simulink model "StPassCmprtMdCrtMdStat"  (R2018b)
settings: Solver=FixedStepDiscrete  StartTime=0.0  StopTime=10.0  FixedStep=0.01  RelTol=1e-3
settings Model: Creator=sn2xws  LastModifiedBy=sn2xws
settings DataIOCC: SaveFormat=StructureWithTime
settings OptimizationCC: DefaultParameterBehavior=Inlined  EnhancedBackFolding=on  PassReuseOutputArgsAs=Individual arguments  ZeroExternalMemoryAtStartup=off  ZeroInternalMemoryAtStartup=off  OptimizeBlockOrder=speed  DifferentSizesBufferReuse=on  OptimizationCustomize=off
settings DebuggingCC: ParameterTunabilityLossMsg=error
settings ModelReferenceCC: ModelReferenceNumInstancesAllowed=Single
settings SFSimCC: MATLABDynamicMemAlloc=off
settings RTWCC: SystemTargetFile=autosar.tlc  GenCodeOnly=on  TemplateMakefile=ert_default_tmf  Description=AUTOSAR  GenerateReport=on  IncludeHyperlinkInReport=on  LaunchReport=on  GenerateTraceInfo=on  GenerateTraceReport=on  GenerateTraceReportSl=on  GenerateTraceReportSf=on  GenerateTraceReportEml=on
settings CodeAppCC: ForceParamTrailComments=on  IgnoreCustomStorageClasses=off  OperatorAnnotations=on  SimulinkDataObjDesc=on  SFDataObjDesc=on  InsertBlockDesc=on
settings STFCustomTargetCC: TargetLangStandard=C99 (ISO)  MultiwordLength=256  ParMdlRefBuildCompliant=on  CompOptLevelCompliant=on  IncludeMdlTerminateFcn=off  CombineOutputUpdateFcns=on  SuppressErrorStatus=on  ERTCustomFileBanners=on  SupportNonFinite=off  SupportComplex=off  SupportContinuousTime=off  SupportNonInlinedSFcns=off  RemoveResetFunc=on  MATLABClassNameForMDSCustomization=Simulink.SoftwareTarget.ERTCustomization  AutosarCompliant=on  UseToolchainInfoCompliant=on  LookupTableObjectStructAxisOrder=2,1,3,4,...  LUTObjectStructOrderEvenSpacing=Size,Table,Breakpoints  SystemTargetFile=autosar.tlc
settings ERTTargetCC: TargetLangStandard=C99 (ISO)  ConcurrentExecutionCompliant=off  IncludeMdlTerminateFcn=off  SuppressErrorStatus=on  SupportNonFinite=off  SupportComplex=off  ModelStepFunctionPrototypeControlCompliant=off  CPPClassGenCompliant=off  AutosarCompliant=on  LookupTableObjectStructAxisOrder=2,1,3,4,...  LUTObjectStructOrderEvenSpacing=Size,Table,Breakpoints  InlinedParameterPlacement=NonHierarchical  ERTCustomFileTemplate=example_file_process.tlc

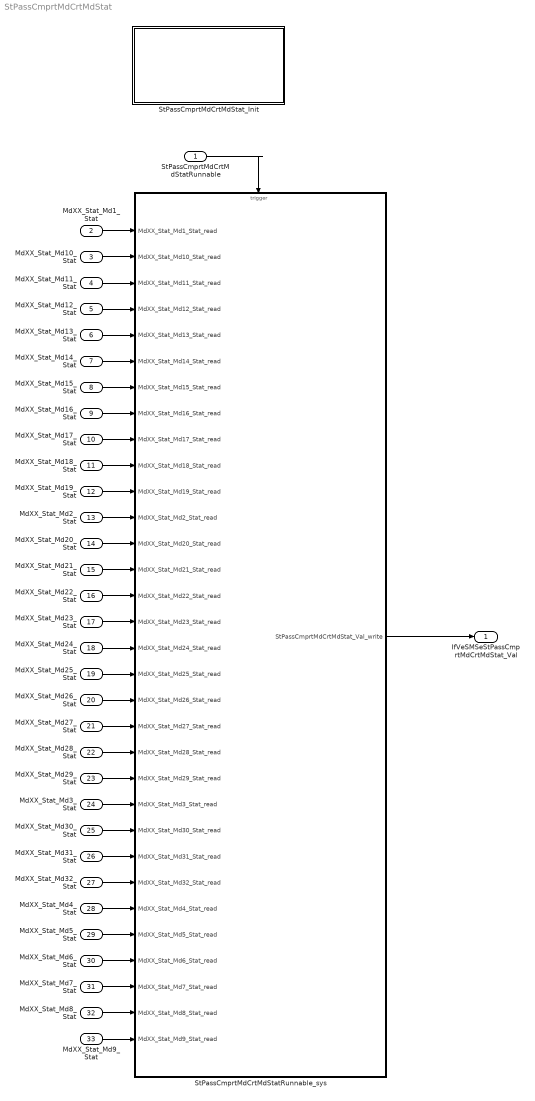
== system StPassCmprtMdCrtMdStat ==
  StPassCmprtMdCrtMdStatRunnable : Inport  SampleTime=0.01  OutputFunctionCall=on
  MdXX_Stat_Md1_Stat : Inport  Port=2  OutDataTypeStr=uint8  PortDimensions=1
  MdXX_Stat_Md10_Stat : Inport  Port=3  OutDataTypeStr=uint8  PortDimensions=1
  MdXX_Stat_Md11_Stat : Inport  Port=4  OutDataTypeStr=uint8  PortDimensions=1
  MdXX_Stat_Md12_Stat : Inport  Port=5  OutDataTypeStr=uint8  PortDimensions=1
  MdXX_Stat_Md13_Stat : Inport  Port=6  OutDataTypeStr=uint8  PortDimensions=1
  MdXX_Stat_Md14_Stat : Inport  Port=7  OutDataTypeStr=uint8  PortDimensions=1
  MdXX_Stat_Md15_Stat : Inport  Port=8  OutDataTypeStr=uint8  PortDimensions=1
  MdXX_Stat_Md16_Stat : Inport  Port=9  OutDataTypeStr=uint8  PortDimensions=1
  MdXX_Stat_Md17_Stat : Inport  Port=10  OutDataTypeStr=uint8  PortDimensions=1
  MdXX_Stat_Md18_Stat : Inport  Port=11  OutDataTypeStr=uint8  PortDimensions=1
  MdXX_Stat_Md19_Stat : Inport  Port=12  OutDataTypeStr=uint8  PortDimensions=1
  MdXX_Stat_Md2_Stat : Inport  Port=13  OutDataTypeStr=uint8  PortDimensions=1
  MdXX_Stat_Md20_Stat : Inport  Port=14  OutDataTypeStr=uint8  PortDimensions=1
  MdXX_Stat_Md21_Stat : Inport  Port=15  OutDataTypeStr=uint8  PortDimensions=1
  MdXX_Stat_Md22_Stat : Inport  Port=16  OutDataTypeStr=uint8  PortDimensions=1
  MdXX_Stat_Md23_Stat : Inport  Port=17  OutDataTypeStr=uint8  PortDimensions=1
  MdXX_Stat_Md24_Stat : Inport  Port=18  OutDataTypeStr=uint8  PortDimensions=1
  MdXX_Stat_Md25_Stat : Inport  Port=19  OutDataTypeStr=uint8  PortDimensions=1
  MdXX_Stat_Md26_Stat : Inport  Port=20  OutDataTypeStr=uint8  PortDimensions=1
  MdXX_Stat_Md27_Stat : Inport  Port=21  OutDataTypeStr=uint8  PortDimensions=1
  MdXX_Stat_Md28_Stat : Inport  Port=22  OutDataTypeStr=uint8  PortDimensions=1
  MdXX_Stat_Md29_Stat : Inport  Port=23  OutDataTypeStr=uint8  PortDimensions=1
  MdXX_Stat_Md3_Stat : Inport  Port=24  OutDataTypeStr=uint8  PortDimensions=1
  MdXX_Stat_Md30_Stat : Inport  Port=25  OutDataTypeStr=uint8  PortDimensions=1
  MdXX_Stat_Md31_Stat : Inport  Port=26  OutDataTypeStr=uint8  PortDimensions=1
  MdXX_Stat_Md32_Stat : Inport  Port=27  OutDataTypeStr=uint8  PortDimensions=1
  MdXX_Stat_Md4_Stat : Inport  Port=28  OutDataTypeStr=uint8  PortDimensions=1
  MdXX_Stat_Md5_Stat : Inport  Port=29  OutDataTypeStr=uint8  PortDimensions=1
  MdXX_Stat_Md6_Stat : Inport  Port=30  OutDataTypeStr=uint8  PortDimensions=1
  MdXX_Stat_Md7_Stat : Inport  Port=31  OutDataTypeStr=uint8  PortDimensions=1
  MdXX_Stat_Md8_Stat : Inport  Port=32  OutDataTypeStr=uint8  PortDimensions=1
  MdXX_Stat_Md9_Stat : Inport  Port=33  OutDataTypeStr=uint8  PortDimensions=1
  StPassCmprtMdCrtMdStatRunnable_sys : Subsystem
  StPassCmprtMdCrtMdStat_Init : Subsystem
  IfVeSMSeStPassCmprtMdCrtMdStat_Val : Outport  OutDataTypeStr=uint8  PortDimensions=1
  wires:
  MdXX_Stat_Md1_Stat/1 -> StPassCmprtMdCrtMdStatRunnable_sys/1(MdXX_Stat_Md1_Stat_read)
  MdXX_Stat_Md10_Stat/1 -> StPassCmprtMdCrtMdStatRunnable_sys/2(MdXX_Stat_Md10_Stat_read)
  MdXX_Stat_Md11_Stat/1 -> StPassCmprtMdCrtMdStatRunnable_sys/3(MdXX_Stat_Md11_Stat_read)
  MdXX_Stat_Md12_Stat/1 -> StPassCmprtMdCrtMdStatRunnable_sys/4(MdXX_Stat_Md12_Stat_read)
  MdXX_Stat_Md13_Stat/1 -> StPassCmprtMdCrtMdStatRunnable_sys/5(MdXX_Stat_Md13_Stat_read)
  MdXX_Stat_Md14_Stat/1 -> StPassCmprtMdCrtMdStatRunnable_sys/6(MdXX_Stat_Md14_Stat_read)
  MdXX_Stat_Md15_Stat/1 -> StPassCmprtMdCrtMdStatRunnable_sys/7(MdXX_Stat_Md15_Stat_read)
  MdXX_Stat_Md16_Stat/1 -> StPassCmprtMdCrtMdStatRunnable_sys/8(MdXX_Stat_Md16_Stat_read)
  MdXX_Stat_Md17_Stat/1 -> StPassCmprtMdCrtMdStatRunnable_sys/9(MdXX_Stat_Md17_Stat_read)
  MdXX_Stat_Md18_Stat/1 -> StPassCmprtMdCrtMdStatRunnable_sys/10(MdXX_Stat_Md18_Stat_read)
  MdXX_Stat_Md19_Stat/1 -> StPassCmprtMdCrtMdStatRunnable_sys/11(MdXX_Stat_Md19_Stat_read)
  MdXX_Stat_Md2_Stat/1 -> StPassCmprtMdCrtMdStatRunnable_sys/12(MdXX_Stat_Md2_Stat_read)
  MdXX_Stat_Md20_Stat/1 -> StPassCmprtMdCrtMdStatRunnable_sys/13(MdXX_Stat_Md20_Stat_read)
  MdXX_Stat_Md21_Stat/1 -> StPassCmprtMdCrtMdStatRunnable_sys/14(MdXX_Stat_Md21_Stat_read)
  MdXX_Stat_Md22_Stat/1 -> StPassCmprtMdCrtMdStatRunnable_sys/15(MdXX_Stat_Md22_Stat_read)
  MdXX_Stat_Md23_Stat/1 -> StPassCmprtMdCrtMdStatRunnable_sys/16(MdXX_Stat_Md23_Stat_read)
  MdXX_Stat_Md24_Stat/1 -> StPassCmprtMdCrtMdStatRunnable_sys/17(MdXX_Stat_Md24_Stat_read)
  MdXX_Stat_Md25_Stat/1 -> StPassCmprtMdCrtMdStatRunnable_sys/18(MdXX_Stat_Md25_Stat_read)
  MdXX_Stat_Md26_Stat/1 -> StPassCmprtMdCrtMdStatRunnable_sys/19(MdXX_Stat_Md26_Stat_read)
  MdXX_Stat_Md27_Stat/1 -> StPassCmprtMdCrtMdStatRunnable_sys/20(MdXX_Stat_Md27_Stat_read)
  MdXX_Stat_Md28_Stat/1 -> StPassCmprtMdCrtMdStatRunnable_sys/21(MdXX_Stat_Md28_Stat_read)
  MdXX_Stat_Md29_Stat/1 -> StPassCmprtMdCrtMdStatRunnable_sys/22(MdXX_Stat_Md29_Stat_read)
  MdXX_Stat_Md3_Stat/1 -> StPassCmprtMdCrtMdStatRunnable_sys/23(MdXX_Stat_Md3_Stat_read)
  MdXX_Stat_Md30_Stat/1 -> StPassCmprtMdCrtMdStatRunnable_sys/24(MdXX_Stat_Md30_Stat_read)
  MdXX_Stat_Md31_Stat/1 -> StPassCmprtMdCrtMdStatRunnable_sys/25(MdXX_Stat_Md31_Stat_read)
  MdXX_Stat_Md32_Stat/1 -> StPassCmprtMdCrtMdStatRunnable_sys/26(MdXX_Stat_Md32_Stat_read)
  MdXX_Stat_Md4_Stat/1 -> StPassCmprtMdCrtMdStatRunnable_sys/27(MdXX_Stat_Md4_Stat_read)
  MdXX_Stat_Md5_Stat/1 -> StPassCmprtMdCrtMdStatRunnable_sys/28(MdXX_Stat_Md5_Stat_read)
  MdXX_Stat_Md6_Stat/1 -> StPassCmprtMdCrtMdStatRunnable_sys/29(MdXX_Stat_Md6_Stat_read)
  MdXX_Stat_Md7_Stat/1 -> StPassCmprtMdCrtMdStatRunnable_sys/30(MdXX_Stat_Md7_Stat_read)
  MdXX_Stat_Md8_Stat/1 -> StPassCmprtMdCrtMdStatRunnable_sys/31(MdXX_Stat_Md8_Stat_read)
  MdXX_Stat_Md9_Stat/1 -> StPassCmprtMdCrtMdStatRunnable_sys/32(MdXX_Stat_Md9_Stat_read)
  StPassCmprtMdCrtMdStatRunnable_sys/1(StPassCmprtMdCrtMdStat_Val_write) -> IfVeSMSeStPassCmprtMdCrtMdStat_Val/1
  StPassCmprtMdCrtMdStatRunnable/1 -> StPassCmprtMdCrtMdStatRunnable_sys/Trigger

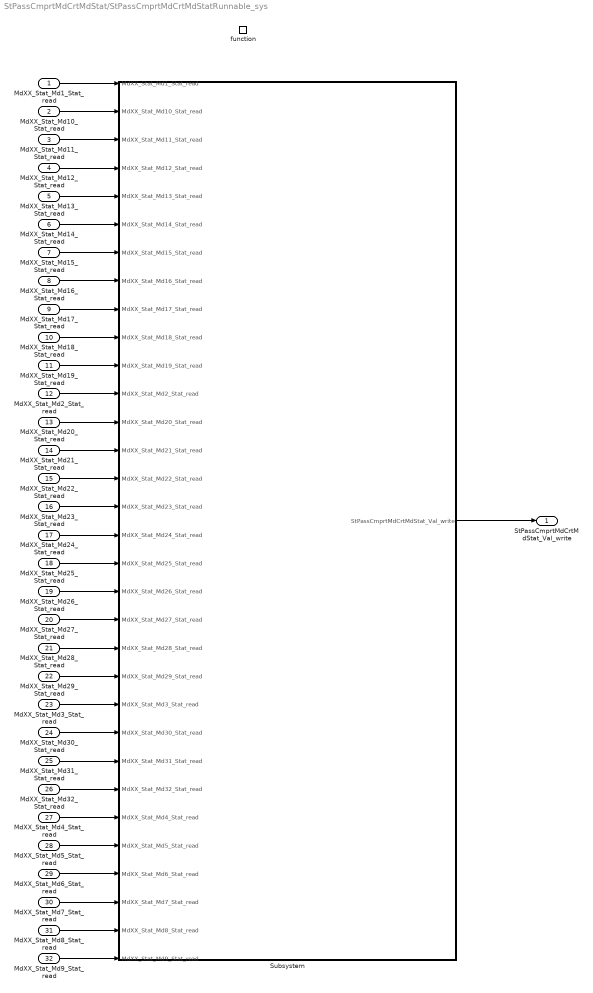
== system StPassCmprtMdCrtMdStat/StPassCmprtMdCrtMdStatRunnable_sys ==
  MdXX_Stat_Md1_Stat_read : Inport
  MdXX_Stat_Md10_Stat_read : Inport  Port=2
  MdXX_Stat_Md11_Stat_read : Inport  Port=3
  MdXX_Stat_Md12_Stat_read : Inport  Port=4
  MdXX_Stat_Md13_Stat_read : Inport  Port=5
  MdXX_Stat_Md14_Stat_read : Inport  Port=6
  MdXX_Stat_Md15_Stat_read : Inport  Port=7
  MdXX_Stat_Md16_Stat_read : Inport  Port=8
  MdXX_Stat_Md17_Stat_read : Inport  Port=9
  MdXX_Stat_Md18_Stat_read : Inport  Port=10
  MdXX_Stat_Md19_Stat_read : Inport  Port=11
  MdXX_Stat_Md2_Stat_read : Inport  Port=12
  MdXX_Stat_Md20_Stat_read : Inport  Port=13
  MdXX_Stat_Md21_Stat_read : Inport  Port=14
  MdXX_Stat_Md22_Stat_read : Inport  Port=15
  MdXX_Stat_Md23_Stat_read : Inport  Port=16
  MdXX_Stat_Md24_Stat_read : Inport  Port=17
  MdXX_Stat_Md25_Stat_read : Inport  Port=18
  MdXX_Stat_Md26_Stat_read : Inport  Port=19
  MdXX_Stat_Md27_Stat_read : Inport  Port=20
  MdXX_Stat_Md28_Stat_read : Inport  Port=21
  MdXX_Stat_Md29_Stat_read : Inport  Port=22
  MdXX_Stat_Md3_Stat_read : Inport  Port=23
  MdXX_Stat_Md30_Stat_read : Inport  Port=24
  MdXX_Stat_Md31_Stat_read : Inport  Port=25
  MdXX_Stat_Md32_Stat_read : Inport  Port=26
  MdXX_Stat_Md4_Stat_read : Inport  Port=27
  MdXX_Stat_Md5_Stat_read : Inport  Port=28
  MdXX_Stat_Md6_Stat_read : Inport  Port=29
  MdXX_Stat_Md7_Stat_read : Inport  Port=30
  MdXX_Stat_Md8_Stat_read : Inport  Port=31
  MdXX_Stat_Md9_Stat_read : Inport  Port=32
  function : TriggerPort  TriggerType=function-call  VariantControl=(inherit)  SampleTimeType=periodic  SampleTime=-1
  Subsystem : Subsystem
  StPassCmprtMdCrtMdStat_Val_write : Outport
      settings: EnsureOutportIsVirtual=on
  wires:
  MdXX_Stat_Md1_Stat_read/1 -> Subsystem/1(MdXX_Stat_Md1_Stat_read)
  MdXX_Stat_Md10_Stat_read/1 -> Subsystem/2(MdXX_Stat_Md10_Stat_read)
  MdXX_Stat_Md11_Stat_read/1 -> Subsystem/3(MdXX_Stat_Md11_Stat_read)
  MdXX_Stat_Md12_Stat_read/1 -> Subsystem/4(MdXX_Stat_Md12_Stat_read)
  MdXX_Stat_Md13_Stat_read/1 -> Subsystem/5(MdXX_Stat_Md13_Stat_read)
  MdXX_Stat_Md14_Stat_read/1 -> Subsystem/6(MdXX_Stat_Md14_Stat_read)
  MdXX_Stat_Md15_Stat_read/1 -> Subsystem/7(MdXX_Stat_Md15_Stat_read)
  MdXX_Stat_Md16_Stat_read/1 -> Subsystem/8(MdXX_Stat_Md16_Stat_read)
  MdXX_Stat_Md17_Stat_read/1 -> Subsystem/9(MdXX_Stat_Md17_Stat_read)
  MdXX_Stat_Md18_Stat_read/1 -> Subsystem/10(MdXX_Stat_Md18_Stat_read)
  MdXX_Stat_Md19_Stat_read/1 -> Subsystem/11(MdXX_Stat_Md19_Stat_read)
  MdXX_Stat_Md2_Stat_read/1 -> Subsystem/12(MdXX_Stat_Md2_Stat_read)
  MdXX_Stat_Md20_Stat_read/1 -> Subsystem/13(MdXX_Stat_Md20_Stat_read)
  MdXX_Stat_Md21_Stat_read/1 -> Subsystem/14(MdXX_Stat_Md21_Stat_read)
  MdXX_Stat_Md22_Stat_read/1 -> Subsystem/15(MdXX_Stat_Md22_Stat_read)
  MdXX_Stat_Md23_Stat_read/1 -> Subsystem/16(MdXX_Stat_Md23_Stat_read)
  MdXX_Stat_Md24_Stat_read/1 -> Subsystem/17(MdXX_Stat_Md24_Stat_read)
  MdXX_Stat_Md25_Stat_read/1 -> Subsystem/18(MdXX_Stat_Md25_Stat_read)
  MdXX_Stat_Md26_Stat_read/1 -> Subsystem/19(MdXX_Stat_Md26_Stat_read)
  MdXX_Stat_Md27_Stat_read/1 -> Subsystem/20(MdXX_Stat_Md27_Stat_read)
  MdXX_Stat_Md28_Stat_read/1 -> Subsystem/21(MdXX_Stat_Md28_Stat_read)
  MdXX_Stat_Md29_Stat_read/1 -> Subsystem/22(MdXX_Stat_Md29_Stat_read)
  MdXX_Stat_Md3_Stat_read/1 -> Subsystem/23(MdXX_Stat_Md3_Stat_read)
  MdXX_Stat_Md30_Stat_read/1 -> Subsystem/24(MdXX_Stat_Md30_Stat_read)
  MdXX_Stat_Md31_Stat_read/1 -> Subsystem/25(MdXX_Stat_Md31_Stat_read)
  MdXX_Stat_Md32_Stat_read/1 -> Subsystem/26(MdXX_Stat_Md32_Stat_read)
  MdXX_Stat_Md4_Stat_read/1 -> Subsystem/27(MdXX_Stat_Md4_Stat_read)
  MdXX_Stat_Md5_Stat_read/1 -> Subsystem/28(MdXX_Stat_Md5_Stat_read)
  MdXX_Stat_Md6_Stat_read/1 -> Subsystem/29(MdXX_Stat_Md6_Stat_read)
  MdXX_Stat_Md7_Stat_read/1 -> Subsystem/30(MdXX_Stat_Md7_Stat_read)
  MdXX_Stat_Md8_Stat_read/1 -> Subsystem/31(MdXX_Stat_Md8_Stat_read)
  MdXX_Stat_Md9_Stat_read/1 -> Subsystem/32(MdXX_Stat_Md9_Stat_read)
  Subsystem/1(StPassCmprtMdCrtMdStat_Val_write) -> StPassCmprtMdCrtMdStat_Val_write/1

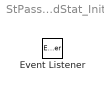
== system StPassCmprtMdCrtMdStat/StPassCmprtMdCrtMdStat_Init ==
  Event Listener : EventListener  EventName=reset

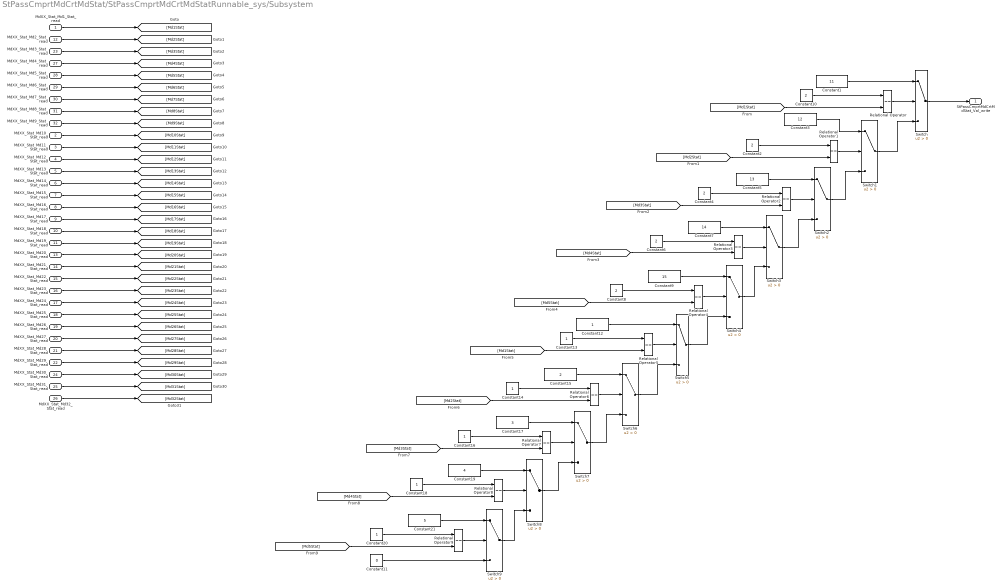
== system StPassCmprtMdCrtMdStat/StPassCmprtMdCrtMdStatRunnable_sys/Subsystem ==
  MdXX_Stat_Md1_Stat_read : Inport
  MdXX_Stat_Md10_Stat_read : Inport  Port=2
  MdXX_Stat_Md11_Stat_read : Inport  Port=3
  MdXX_Stat_Md12_Stat_read : Inport  Port=4
  MdXX_Stat_Md13_Stat_read : Inport  Port=5
  MdXX_Stat_Md14_Stat_read : Inport  Port=6
  MdXX_Stat_Md15_Stat_read : Inport  Port=7
  MdXX_Stat_Md16_Stat_read : Inport  Port=8
  MdXX_Stat_Md17_Stat_read : Inport  Port=9
  MdXX_Stat_Md18_Stat_read : Inport  Port=10
  MdXX_Stat_Md19_Stat_read : Inport  Port=11
  MdXX_Stat_Md2_Stat_read : Inport  Port=12
  MdXX_Stat_Md20_Stat_read : Inport  Port=13
  MdXX_Stat_Md21_Stat_read : Inport  Port=14
  MdXX_Stat_Md22_Stat_read : Inport  Port=15
  MdXX_Stat_Md23_Stat_read : Inport  Port=16
  MdXX_Stat_Md24_Stat_read : Inport  Port=17
  MdXX_Stat_Md25_Stat_read : Inport  Port=18
  MdXX_Stat_Md26_Stat_read : Inport  Port=19
  MdXX_Stat_Md27_Stat_read : Inport  Port=20
  MdXX_Stat_Md28_Stat_read : Inport  Port=21
  MdXX_Stat_Md29_Stat_read : Inport  Port=22
  MdXX_Stat_Md3_Stat_read : Inport  Port=23
  MdXX_Stat_Md30_Stat_read : Inport  Port=24
  MdXX_Stat_Md31_Stat_read : Inport  Port=25
  MdXX_Stat_Md32_Stat_read : Inport  Port=26
  MdXX_Stat_Md4_Stat_read : Inport  Port=27
  MdXX_Stat_Md5_Stat_read : Inport  Port=28
  MdXX_Stat_Md6_Stat_read : Inport  Port=29
  MdXX_Stat_Md7_Stat_read : Inport  Port=30
  MdXX_Stat_Md8_Stat_read : Inport  Port=31
  MdXX_Stat_Md9_Stat_read : Inport  Port=32
  Constant1 : Constant  Value=11  OutDataTypeStr=uint8
  Constant{2,4,6,8,10,15} (6 alike) : Constant  Value=2  OutDataTypeStr=uint8
  Constant11 : Constant  Value=0  OutDataTypeStr=uint8
  Constant{12..14,16,18,20} (6 alike) : Constant  OutDataTypeStr=uint8
  Constant17 : Constant  Value=3  OutDataTypeStr=uint8
  Constant19 : Constant  Value=4  OutDataTypeStr=uint8
  Constant21 : Constant  Value=5  OutDataTypeStr=uint8
  Constant3 : Constant  Value=12  OutDataTypeStr=uint8
  Constant5 : Constant  Value=13  OutDataTypeStr=uint8
  Constant7 : Constant  Value=14  OutDataTypeStr=uint8
  Constant9 : Constant  Value=15  OutDataTypeStr=uint8
  Relational Operator{,1..9} (10 alike) : RelationalOperator  Operator===  OutDataTypeStr=boolean  RndMeth=Simplest
  Switch{,1..9} (10 alike) : Switch  Criteria=u2 > Threshold
  StPassCmprtMdCrtMdStat_Val_write : Outport
      settings: EnsureOutportIsVirtual=on
  wires:
  Constant11/1 -> Switch9/3
  [Md1Stat] -> Relational Operator5/2
  Constant3/1 -> Switch1/1
  Constant1/1 -> Switch/1
  Relational Operator4/1 -> Switch4/2
  Constant12/1 -> Switch5/1
  Switch5/1 -> Switch4/3
  Switch9/1 -> Switch8/3
  [Md3Stat] -> Relational Operator2/2
  Constant15/1 -> Switch6/1
  Constant14/1 -> Relational Operator6/1
  Relational Operator5/1 -> Switch5/2
  Constant13/1 -> Relational Operator5/1
  Relational Operator9/1 -> Switch9/2
  Relational Operator7/1 -> Switch7/2
  Constant5/1 -> Switch2/1
  Switch6/1 -> Switch5/3
  Constant16/1 -> Relational Operator7/1
  [Md5Stat] -> Relational Operator9/2
  Switch1/1 -> Switch/3
  Relational Operator6/1 -> Switch6/2
  [Md4Stat] -> Relational Operator8/2
  Constant21/1 -> Switch9/1
  Relational Operator2/1 -> Switch2/2
  Constant4/1 -> Relational Operator2/1
  Constant19/1 -> Switch8/1
  Constant2/1 -> Relational Operator1/1
  [Md2Stat] -> Relational Operator6/2
  Constant8/1 -> Relational Operator4/1
  Switch8/1 -> Switch7/3
  Relational Operator/1 -> Switch/2
  Constant20/1 -> Relational Operator9/1
  Switch7/1 -> Switch6/3
  [Md5Stat] -> Relational Operator4/2
  Constant6/1 -> Relational Operator3/1
  Switch/1 -> StPassCmprtMdCrtMdStat_Val_write/1
  [Md1Stat] -> Relational Operator/2
  Constant18/1 -> Relational Operator8/1
  Switch3/1 -> Switch2/3
  Switch4/1 -> Switch3/3
  [Md2Stat] -> Relational Operator1/2
  Constant9/1 -> Switch4/1
  Constant17/1 -> Switch7/1
  [Md3Stat] -> Relational Operator7/2
  Relational Operator3/1 -> Switch3/2
  Constant7/1 -> Switch3/1
  Relational Operator1/1 -> Switch1/2
  [Md4Stat] -> Relational Operator3/2
  Relational Operator8/1 -> Switch8/2
  Constant10/1 -> Relational Operator/1
  Switch2/1 -> Switch1/3
  MdXX_Stat_Md1_Stat_read/1 -> [Md1Stat]
  MdXX_Stat_Md2_Stat_read/1 -> [Md2Stat]
  MdXX_Stat_Md3_Stat_read/1 -> [Md3Stat]
  MdXX_Stat_Md4_Stat_read/1 -> [Md4Stat]
  MdXX_Stat_Md5_Stat_read/1 -> [Md5Stat]
  MdXX_Stat_Md6_Stat_read/1 -> [Md6Stat]
  MdXX_Stat_Md7_Stat_read/1 -> [Md7Stat]
  MdXX_Stat_Md8_Stat_read/1 -> [Md8Stat]
  MdXX_Stat_Md9_Stat_read/1 -> [Md9Stat]
  MdXX_Stat_Md10_Stat_read/1 -> [Md10Stat]
  MdXX_Stat_Md11_Stat_read/1 -> [Md11Stat]
  MdXX_Stat_Md12_Stat_read/1 -> [Md12Stat]
  MdXX_Stat_Md13_Stat_read/1 -> [Md13Stat]
  MdXX_Stat_Md14_Stat_read/1 -> [Md14Stat]
  MdXX_Stat_Md15_Stat_read/1 -> [Md15Stat]
  MdXX_Stat_Md16_Stat_read/1 -> [Md16Stat]
  MdXX_Stat_Md17_Stat_read/1 -> [Md17Stat]
  MdXX_Stat_Md18_Stat_read/1 -> [Md18Stat]
  MdXX_Stat_Md19_Stat_read/1 -> [Md19Stat]
  MdXX_Stat_Md20_Stat_read/1 -> [Md20Stat]
  MdXX_Stat_Md21_Stat_read/1 -> [Md21Stat]
  MdXX_Stat_Md22_Stat_read/1 -> [Md22Stat]
  MdXX_Stat_Md23_Stat_read/1 -> [Md23Stat]
  MdXX_Stat_Md24_Stat_read/1 -> [Md24Stat]
  MdXX_Stat_Md25_Stat_read/1 -> [Md25Stat]
  MdXX_Stat_Md26_Stat_read/1 -> [Md26Stat]
  MdXX_Stat_Md27_Stat_read/1 -> [Md27Stat]
  MdXX_Stat_Md28_Stat_read/1 -> [Md28Stat]
  MdXX_Stat_Md29_Stat_read/1 -> [Md29Stat]
  MdXX_Stat_Md30_Stat_read/1 -> [Md30Stat]
  MdXX_Stat_Md32_Stat_read/1 -> [Md32Stat]
  MdXX_Stat_Md31_Stat_read/1 -> [Md31Stat]
